simulink model "cart_pi_step_dis_sim"  (R2013a)
settings: Solver=ode4  StartTime=0.0  StopTime=t_end  FixedStep=0.001  RelTol=1e-3
values from neighbouring files (symbols this model uses):
  ac = 6.25    [p1c62_ex1_cart_p_step.m]    (also in p1c62_ex2_cart_pi_ramp.m; p1c62_ex3_cart_p_step_dis.m; p1c62_ex4_cart_pi_step_dis.m)
  bc = 4.36    [p1c62_ex1_cart_p_step.m]    (also in p1c62_ex2_cart_pi_ramp.m; p1c62_ex3_cart_p_step_dis.m; p1c62_ex4_cart_pi_step_dis.m)
  d0 = 3    [p1c62_ex3_cart_p_step_dis.m]    (also in p1c62_ex4_cart_pi_step_dis.m; p1c63_ex5_cdip_lqr_servo.m = 5)
  kI = 15    [p1c62_ex2_cart_pi_ramp.m]    (also in p1c62_ex3_cart_p_step_dis.m = 0; p1c62_ex4_cart_pi_step_dis.m)
  kP = 10    [p1c62_ex1_cart_p_step.m]    (also in p1c62_ex2_cart_pi_ramp.m; p1c62_ex3_cart_p_step_dis.m; p1c62_ex4_cart_pi_step_dis.m)
  r0 = 0.5    [p1c62_ex1_cart_p_step.m]    (also in p1c62_ex2_cart_pi_ramp.m = 0.1; p1c62_ex3_cart_p_step_dis.m; p1c62_ex4_cart_pi_step_dis.m; p1c63_ex5_cdip_lqr_servo.m)
  t_dis = 2.5    [p1c62_ex3_cart_p_step_dis.m]    (also in p1c62_ex4_cart_pi_step_dis.m; p1c63_ex5_cdip_lqr_servo.m)
settings Model: Creator=kawata  LastModifiedBy=kawata

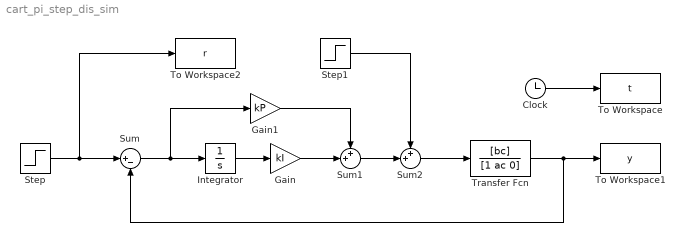
== system cart_pi_step_dis_sim ==
  Clock : Clock
  Gain : Gain  Gain=kI
  Gain1 : Gain  Gain=kP
  Integrator : Integrator
  Step : Step  Time=0  After=r0  SampleTime=0
  Step1 : Step  Time=t_dis  After=d0  SampleTime=0
  Sum : Sum  Inputs=|+-
  Sum1 : Sum  Inputs=++|
  Sum2 : Sum  Inputs=++|
  To Workspace : ToWorkspace  VariableName=t  SampleTime=-1
  To Workspace1 : ToWorkspace  VariableName=y  SampleTime=-1
  To Workspace2 : ToWorkspace  VariableName=r  SampleTime=-1
  Transfer Fcn : TransferFcn  Numerator=[bc]  Denominator=[1 ac 0]
  wires:
  Step/1 -> To Workspace2/1, Sum/1
  Sum/1 -> Gain1/1, Integrator/1
  Integrator/1 -> Gain/1
  Gain/1 -> Sum1/2
  Gain1/1 -> Sum1/1
  Transfer Fcn/1 -> Sum/2, To Workspace1/1
  Clock/1 -> To Workspace/1
  Sum1/1 -> Sum2/2
  Sum2/1 -> Transfer Fcn/1
  Step1/1 -> Sum2/1
